simulink library "DiSC_ToolboxOpal_V12"  (R2012b)
settings: Solver=ode45  StartTime=0.0  StopTime=10.0  RelTol=1e-3
undefined symbols (not defined in the file or in its folder): SamplingTime
(part 3 of 5)

== system DiSC_ToolboxOpal_V12/scAsset ==
  In1 : Inport
  In2 : Inport  Port=2
  In3 : Inport  Port=3
  In4 : Inport  Port=4
  MATLAB Function : MATLAB Function  TreatAsAtomicUnit=on
  Out1 : Outport
  wires:
  MATLAB Function/1(q) -> Out1/1
  In4/1 -> MATLAB Function/4(t)
  In1/1 -> MATLAB Function/1(v)
  In2/1 -> MATLAB Function/2(qRef)
  In3/1 -> MATLAB Function/3(vRef)

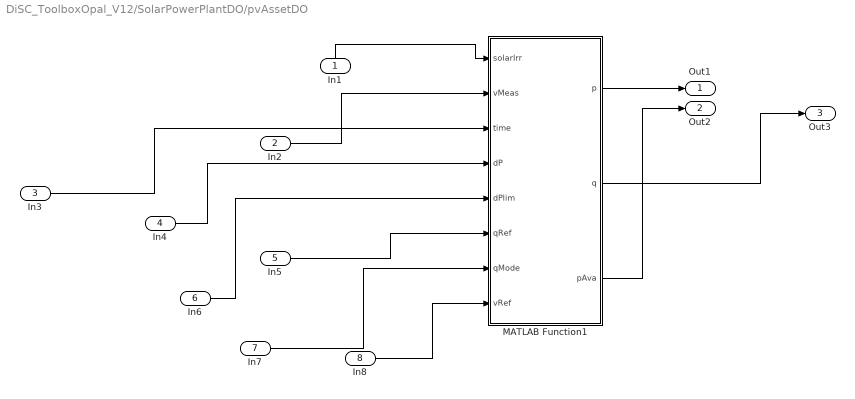
== system DiSC_ToolboxOpal_V12/SolarPowerPlantDO/pvAssetDO ==
  In1 : Inport
  In2 : Inport  Port=2
  In3 : Inport  Port=3
  In4 : Inport  Port=4
  In5 : Inport  Port=5
  In6 : Inport  Port=6
  In7 : Inport  Port=7
  In8 : Inport  Port=8
  MATLAB Function1 : MATLAB Function  TreatAsAtomicUnit=on
  Out1 : Outport
  Out2 : Outport  Port=2
  Out3 : Outport  Port=3
  wires:
  MATLAB Function1/3(pAva) -> Out2/1
  In5/1 -> MATLAB Function1/6(qRef)
  MATLAB Function1/1(p) -> Out1/1
  In2/1 -> MATLAB Function1/2(vMeas)
  In4/1 -> MATLAB Function1/4(dP)
  In6/1 -> MATLAB Function1/5(dPlim)
  In3/1 -> MATLAB Function1/3(time)
  In1/1 -> MATLAB Function1/1(solarIrr)
  MATLAB Function1/2(q) -> Out3/1
  In8/1 -> MATLAB Function1/8(vRef)
  In7/1 -> MATLAB Function1/7(qMode)

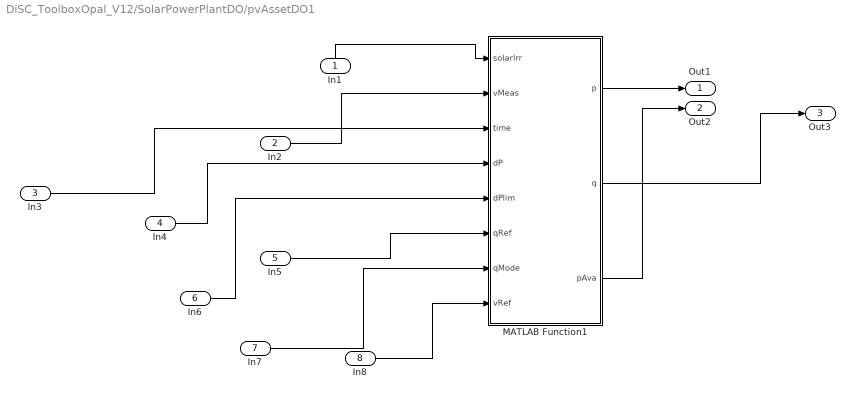
== system DiSC_ToolboxOpal_V12/SolarPowerPlantDO/pvAssetDO1 ==
  In1 : Inport
  In2 : Inport  Port=2
  In3 : Inport  Port=3
  In4 : Inport  Port=4
  In5 : Inport  Port=5
  In6 : Inport  Port=6
  In7 : Inport  Port=7
  In8 : Inport  Port=8
  MATLAB Function1 : MATLAB Function  TreatAsAtomicUnit=on
  Out1 : Outport
  Out2 : Outport  Port=2
  Out3 : Outport  Port=3
  wires:
  MATLAB Function1/3(pAva) -> Out2/1
  In5/1 -> MATLAB Function1/6(qRef)
  MATLAB Function1/1(p) -> Out1/1
  In2/1 -> MATLAB Function1/2(vMeas)
  In4/1 -> MATLAB Function1/4(dP)
  In6/1 -> MATLAB Function1/5(dPlim)
  In3/1 -> MATLAB Function1/3(time)
  In1/1 -> MATLAB Function1/1(solarIrr)
  MATLAB Function1/2(q) -> Out3/1
  In8/1 -> MATLAB Function1/8(vRef)
  In7/1 -> MATLAB Function1/7(qMode)

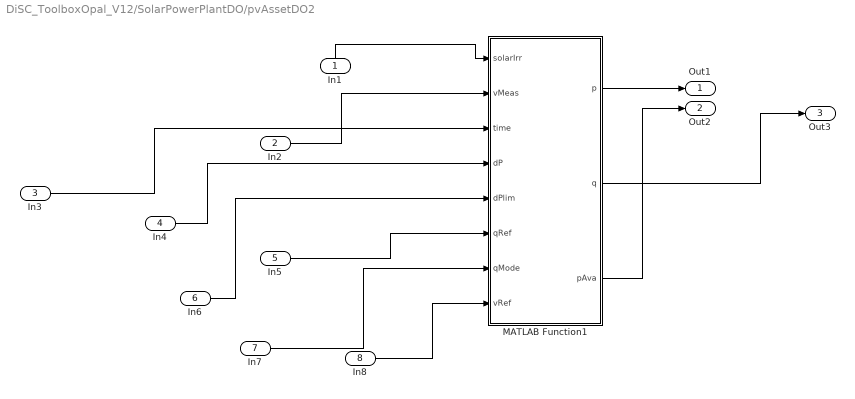
== system DiSC_ToolboxOpal_V12/SolarPowerPlantDO/pvAssetDO2 ==
  In1 : Inport
  In2 : Inport  Port=2
  In3 : Inport  Port=3
  In4 : Inport  Port=4
  In5 : Inport  Port=5
  In6 : Inport  Port=6
  In7 : Inport  Port=7
  In8 : Inport  Port=8
  MATLAB Function1 : MATLAB Function  TreatAsAtomicUnit=on
  Out1 : Outport
  Out2 : Outport  Port=2
  Out3 : Outport  Port=3
  wires:
  MATLAB Function1/3(pAva) -> Out2/1
  In5/1 -> MATLAB Function1/6(qRef)
  MATLAB Function1/1(p) -> Out1/1
  In2/1 -> MATLAB Function1/2(vMeas)
  In4/1 -> MATLAB Function1/4(dP)
  In6/1 -> MATLAB Function1/5(dPlim)
  In3/1 -> MATLAB Function1/3(time)
  In1/1 -> MATLAB Function1/1(solarIrr)
  MATLAB Function1/2(q) -> Out3/1
  In8/1 -> MATLAB Function1/8(vRef)
  In7/1 -> MATLAB Function1/7(qMode)

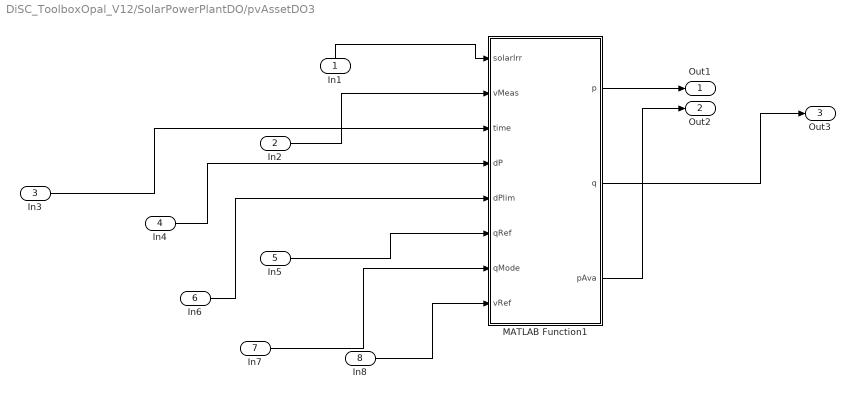
== system DiSC_ToolboxOpal_V12/SolarPowerPlantDO/pvAssetDO3 ==
  In1 : Inport
  In2 : Inport  Port=2
  In3 : Inport  Port=3
  In4 : Inport  Port=4
  In5 : Inport  Port=5
  In6 : Inport  Port=6
  In7 : Inport  Port=7
  In8 : Inport  Port=8
  MATLAB Function1 : MATLAB Function  TreatAsAtomicUnit=on
  Out1 : Outport
  Out2 : Outport  Port=2
  Out3 : Outport  Port=3
  wires:
  MATLAB Function1/3(pAva) -> Out2/1
  In5/1 -> MATLAB Function1/6(qRef)
  MATLAB Function1/1(p) -> Out1/1
  In2/1 -> MATLAB Function1/2(vMeas)
  In4/1 -> MATLAB Function1/4(dP)
  In6/1 -> MATLAB Function1/5(dPlim)
  In3/1 -> MATLAB Function1/3(time)
  In1/1 -> MATLAB Function1/1(solarIrr)
  MATLAB Function1/2(q) -> Out3/1
  In8/1 -> MATLAB Function1/8(vRef)
  In7/1 -> MATLAB Function1/7(qMode)

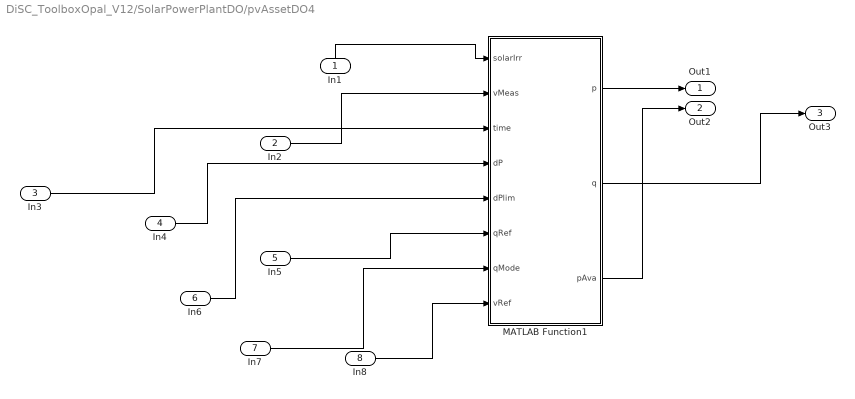
== system DiSC_ToolboxOpal_V12/SolarPowerPlantDO/pvAssetDO4 ==
  In1 : Inport
  In2 : Inport  Port=2
  In3 : Inport  Port=3
  In4 : Inport  Port=4
  In5 : Inport  Port=5
  In6 : Inport  Port=6
  In7 : Inport  Port=7
  In8 : Inport  Port=8
  MATLAB Function1 : MATLAB Function  TreatAsAtomicUnit=on
  Out1 : Outport
  Out2 : Outport  Port=2
  Out3 : Outport  Port=3
  wires:
  MATLAB Function1/3(pAva) -> Out2/1
  In5/1 -> MATLAB Function1/6(qRef)
  MATLAB Function1/1(p) -> Out1/1
  In2/1 -> MATLAB Function1/2(vMeas)
  In4/1 -> MATLAB Function1/4(dP)
  In6/1 -> MATLAB Function1/5(dPlim)
  In3/1 -> MATLAB Function1/3(time)
  In1/1 -> MATLAB Function1/1(solarIrr)
  MATLAB Function1/2(q) -> Out3/1
  In8/1 -> MATLAB Function1/8(vRef)
  In7/1 -> MATLAB Function1/7(qMode)

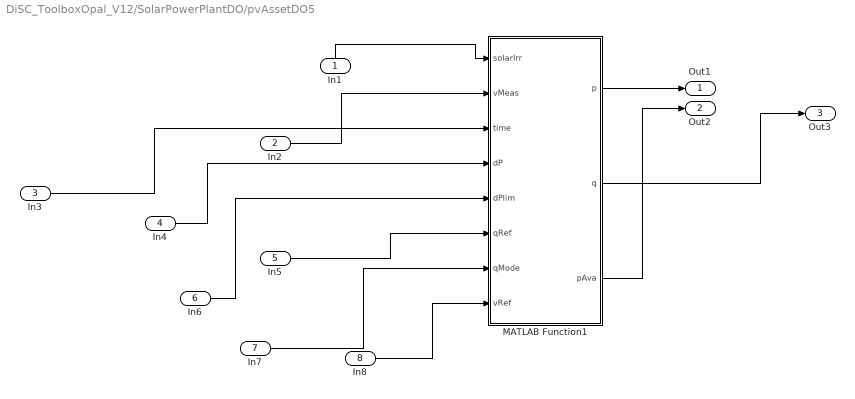
== system DiSC_ToolboxOpal_V12/SolarPowerPlantDO/pvAssetDO5 ==
  In1 : Inport
  In2 : Inport  Port=2
  In3 : Inport  Port=3
  In4 : Inport  Port=4
  In5 : Inport  Port=5
  In6 : Inport  Port=6
  In7 : Inport  Port=7
  In8 : Inport  Port=8
  MATLAB Function1 : MATLAB Function  TreatAsAtomicUnit=on
  Out1 : Outport
  Out2 : Outport  Port=2
  Out3 : Outport  Port=3
  wires:
  MATLAB Function1/3(pAva) -> Out2/1
  In5/1 -> MATLAB Function1/6(qRef)
  MATLAB Function1/1(p) -> Out1/1
  In2/1 -> MATLAB Function1/2(vMeas)
  In4/1 -> MATLAB Function1/4(dP)
  In6/1 -> MATLAB Function1/5(dPlim)
  In3/1 -> MATLAB Function1/3(time)
  In1/1 -> MATLAB Function1/1(solarIrr)
  MATLAB Function1/2(q) -> Out3/1
  In8/1 -> MATLAB Function1/8(vRef)
  In7/1 -> MATLAB Function1/7(qMode)

== system DiSC_ToolboxOpal_V12/WindPowerPlant/wtAssetDO ==
  In1 : Inport
  In2 : Inport  Port=2
  In3 : Inport  Port=3
  In4 : Inport  Port=4
  In5 : Inport  Port=5
  In6 : Inport  Port=6
  In7 : Inport  Port=7
  In8 : Inport  Port=8
  MATLAB Function : MATLAB Function  TreatAsAtomicUnit=on
  Out1 : Outport
  Out2 : Outport  Port=2
  Out3 : Outport  Port=3
  wires:
  In1/1 -> MATLAB Function/1(wind)
  MATLAB Function/3(pAva) -> Out2/1
  In4/1 -> MATLAB Function/4(dPlim)
  MATLAB Function/2(q) -> Out3/1
  In2/1 -> MATLAB Function/2(vMeas)
  In3/1 -> MATLAB Function/3(dP)
  MATLAB Function/1(p) -> Out1/1
  In7/1 -> MATLAB Function/7(vRef)
  In6/1 -> MATLAB Function/6(qMode)
  In5/1 -> MATLAB Function/5(qRef)
  In8/1 -> MATLAB Function/8(time)

== system DiSC_ToolboxOpal_V12/WindPowerPlant/wtAssetDO1 ==
  In1 : Inport
  In2 : Inport  Port=2
  In3 : Inport  Port=3
  In4 : Inport  Port=4
  In5 : Inport  Port=5
  In6 : Inport  Port=6
  In7 : Inport  Port=7
  In8 : Inport  Port=8
  MATLAB Function : MATLAB Function  TreatAsAtomicUnit=on
  Out1 : Outport
  Out2 : Outport  Port=2
  Out3 : Outport  Port=3
  wires:
  In1/1 -> MATLAB Function/1(wind)
  MATLAB Function/3(pAva) -> Out2/1
  In4/1 -> MATLAB Function/4(dPlim)
  MATLAB Function/2(q) -> Out3/1
  In2/1 -> MATLAB Function/2(vMeas)
  In3/1 -> MATLAB Function/3(dP)
  MATLAB Function/1(p) -> Out1/1
  In7/1 -> MATLAB Function/7(vRef)
  In6/1 -> MATLAB Function/6(qMode)
  In5/1 -> MATLAB Function/5(qRef)
  In8/1 -> MATLAB Function/8(time)

== system DiSC_ToolboxOpal_V12/WindPowerPlant/wtAssetDO2 ==
  In1 : Inport
  In2 : Inport  Port=2
  In3 : Inport  Port=3
  In4 : Inport  Port=4
  In5 : Inport  Port=5
  In6 : Inport  Port=6
  In7 : Inport  Port=7
  In8 : Inport  Port=8
  MATLAB Function : MATLAB Function  TreatAsAtomicUnit=on
  Out1 : Outport
  Out2 : Outport  Port=2
  Out3 : Outport  Port=3
  wires:
  In1/1 -> MATLAB Function/1(wind)
  MATLAB Function/3(pAva) -> Out2/1
  In4/1 -> MATLAB Function/4(dPlim)
  MATLAB Function/2(q) -> Out3/1
  In2/1 -> MATLAB Function/2(vMeas)
  In3/1 -> MATLAB Function/3(dP)
  MATLAB Function/1(p) -> Out1/1
  In7/1 -> MATLAB Function/7(vRef)
  In6/1 -> MATLAB Function/6(qMode)
  In5/1 -> MATLAB Function/5(qRef)
  In8/1 -> MATLAB Function/8(time)

== system DiSC_ToolboxOpal_V12/WindPowerPlant/wtAssetDO3 ==
  In1 : Inport
  In2 : Inport  Port=2
  In3 : Inport  Port=3
  In4 : Inport  Port=4
  In5 : Inport  Port=5
  In6 : Inport  Port=6
  In7 : Inport  Port=7
  In8 : Inport  Port=8
  MATLAB Function : MATLAB Function  TreatAsAtomicUnit=on
  Out1 : Outport
  Out2 : Outport  Port=2
  Out3 : Outport  Port=3
  wires:
  In1/1 -> MATLAB Function/1(wind)
  MATLAB Function/3(pAva) -> Out2/1
  In4/1 -> MATLAB Function/4(dPlim)
  MATLAB Function/2(q) -> Out3/1
  In2/1 -> MATLAB Function/2(vMeas)
  In3/1 -> MATLAB Function/3(dP)
  MATLAB Function/1(p) -> Out1/1
  In7/1 -> MATLAB Function/7(vRef)
  In6/1 -> MATLAB Function/6(qMode)
  In5/1 -> MATLAB Function/5(qRef)
  In8/1 -> MATLAB Function/8(time)

== system DiSC_ToolboxOpal_V12/WindPowerPlant/wtAssetDO4 ==
  In1 : Inport
  In2 : Inport  Port=2
  In3 : Inport  Port=3
  In4 : Inport  Port=4
  In5 : Inport  Port=5
  In6 : Inport  Port=6
  In7 : Inport  Port=7
  In8 : Inport  Port=8
  MATLAB Function : MATLAB Function  TreatAsAtomicUnit=on
  Out1 : Outport
  Out2 : Outport  Port=2
  Out3 : Outport  Port=3
  wires:
  In1/1 -> MATLAB Function/1(wind)
  MATLAB Function/3(pAva) -> Out2/1
  In4/1 -> MATLAB Function/4(dPlim)
  MATLAB Function/2(q) -> Out3/1
  In2/1 -> MATLAB Function/2(vMeas)
  In3/1 -> MATLAB Function/3(dP)
  MATLAB Function/1(p) -> Out1/1
  In7/1 -> MATLAB Function/7(vRef)
  In6/1 -> MATLAB Function/6(qMode)
  In5/1 -> MATLAB Function/5(qRef)
  In8/1 -> MATLAB Function/8(time)

== system DiSC_ToolboxOpal_V12/WindPowerPlant/wtAssetDO5 ==
  In1 : Inport
  In2 : Inport  Port=2
  In3 : Inport  Port=3
  In4 : Inport  Port=4
  In5 : Inport  Port=5
  In6 : Inport  Port=6
  In7 : Inport  Port=7
  In8 : Inport  Port=8
  MATLAB Function : MATLAB Function  TreatAsAtomicUnit=on
  Out1 : Outport
  Out2 : Outport  Port=2
  Out3 : Outport  Port=3
  wires:
  In1/1 -> MATLAB Function/1(wind)
  MATLAB Function/3(pAva) -> Out2/1
  In4/1 -> MATLAB Function/4(dPlim)
  MATLAB Function/2(q) -> Out3/1
  In2/1 -> MATLAB Function/2(vMeas)
  In3/1 -> MATLAB Function/3(dP)
  MATLAB Function/1(p) -> Out1/1
  In7/1 -> MATLAB Function/7(vRef)
  In6/1 -> MATLAB Function/6(qMode)
  In5/1 -> MATLAB Function/5(qRef)
  In8/1 -> MATLAB Function/8(time)

== matlab function DiSC_ToolboxOpal_V12/ElectricVehicle/MATLAB Function ==
  data: day input; p output; vMeas input; pRef input; pMode input; qRef input; qMode input; vRef input; time input; seed input; q output; e output; away output
function [p,q,e,away] = evAssetDO(day,vMeas,pRef,pMode,qRef,qMode,vRef,time,seed)
%#codegen
  % evAsset implements a simple electrical vehical mobility- and battery model in Simulink.
    %   The active power consumption of the battery charging cycle can be
    %   controlled when ever the electrical vehical is available at
    %   a household charging spot.
    %   To simulate when the electrical vehical is available data from the
    %   National Travel Survey from Great Britain is used.
    %
    %   To model the battery a simple first order model of an energy
    %   storages is used. The batterys state of charges, when arriving at a
    %   charging station/spot, is dependent on the trip the car has conducted.
    %
    %
    % Revision:
    % 16-07-2014, C.E. Sloth and R. Pedersen, Aalborg University. Notes:
    % 29-11-2014, R. Olsen/M. Kemal, Aalborg University (Simulink)
    % 20-06-2015, F. Iov/M. Kemal, Aalborg University (Simulink toolbox for OPAL)
            % Input:
            %   - k [-], is the sample number.
            %   - day [day number], is the day of the year 1-365.
            %   - v [-], is the voltage at the connection point.
            %   - pRef [W], is the reference to active power.
            %   - qRef [VAR], is the reference to reactive power.
            %   - vRef [V], is the voltage reference.
            %
            % Output:
            %   - p [W], is the active power output.
            %   - q [VAR], is the reactive power output.
            %   - e [J], is the EV batery energy level.
            %   - away [-]. Indicates if the EV is available for charging.
            
            % If day changes calculate when EV is away from home and how
            % much the state of charge has changed.
            
        %properties    
        param.vBase = 20e3;               % Voltage base [V].
        param.pRated = 6e6;               % Rated output power [W].
        param.sMax = 3e6;                 % Maximum apparent power [VA].
        param.pRate = 1000;                 % Constraint on power rate of change [W/s].
        param.PF = 1;                     % Power factor [-].
        param.a = 1;                      % Drain rate of battery [-].
        param.eta = 1;                    % Efficiency of battery [-].
        param.avgMileage = 2;             % Average mileage [% battery/mile].
        param.eRated = 65e3*60*60;        % Battery capacity [J].
        param.Ts = 60;  
        
       %variables
       persistent var;
       if isempty(var) 
        var.eOld = 0;                   % Place holder for battery state [J].
        var.pOld = 0;                   % Power consumption last sample [W].
        var.pMode = 0;                  % Indicates which control mode the charging of the EV is in [-].
        var.qMode = 0;                  % Reactive power control mode [-].
        
        % Modified data based on Table NTS0503
        var.toEducation = [0 0 0 0 0 0 0 7 40 2 1 0 0 0 0 0 0 0 0 0 0 0 0 0];
        var.fromEducation = [0 0 0 0 0 0 0 0 0 0 0 1 2 2 3 32 5 2 1 0 0 0 0 0];
        var.toShopping =    [0 0 0 0 0 0 0 1 2 5 7 7 6 4.5 4.5 3 3 2 2 2 1 0 0 0];
        var.fromShopping =  [0 0 0 0 0 0 0 0 1 3 5 6 5 5 5 5 4 4 3 2 1 1 0 0];
        var.toCommute =   [0 0 0 0 0 3 7 16 15 4 2 2 1 0 0 0 0 0 0 0 0 0 0 0];
        var.fromCommute = [0 0 0 0 0 0 0 0 0 0 0 0 2 3 3 4 9 15 7 2 2 1 1 1];
        var.businessStart = [0 0 0 0 0.5 1 3 7 10 8 7 7 7 7 7 8 9 8 4 2 2 1 1 0.5];
        var.toBusiness =   [0 0 0 0 0.5 1 3 7 10 8 6 5 3.5 2 2 1 1 0 0 0 0 0 0 0];
        var.fromBusiness = [0 0 0 0 0   0 0 0 0  0 1 2 3.5 5 5 7 8 8 4 2 2 1 1 0.5];
        var.toEscortEducation =   [0 0 0 0 0 0 0 3 36 7 0 2 2 0 0 0 0 0 0 0 0 0 0 0];
        var.fromEscortEducation = [0 0 0 0 0 0 0 0 0 0 0 0 0 1 9 33 4 2 1 0 0 0 0 0];
        var.toOtherPersonal =   [0 0 0 0 0 0 1 4 8 8 7 7 6 4 2 1 1 1 0 0 0 0 0 0];
        var.fromOtherPersonal = [0 0 0 0 0 0 0 0 0 0 1 1 2 3 5 7 8 7 6 4 2 2 1 1];
        var.toVisit =   [0 0 0 0 0 0 1 1 2 4 5 6 6 5 4 4 3 3 3 2 1 0 0 0];
        var.fromVisit = [0 0 0 0 0 0 0 0 0 0 0 0 0 1 2 4 5 6 7 8 5 5 4 3];
        var.toHoliday =    [0 0 0 0 0 0 2 4 5 7 8 6 3 3 3 2 2 2 2 1 0 0 0 0];
        var.fromHoliday =  [0 0 0 0 0 0 0 0 0 0 1 3 3 4 5 7 7 5 5 4 3 2 1 1];
        
        % CDFs of mobility model
        var.toCommutingCDF=zeros(1,24);
        var.fromCommutingCDF=zeros(1,24);
        var.toBusinessCDF=zeros(1,24);
        var.fromBusinessCDF=zeros(1,24);
        var.toEducationCDF=zeros(1,24);
        var.fromEducationCDF=zeros(1,24);
        var.toEscortEducationCDF=zeros(1,24);
        var.fromEscortEducationCDF=zeros(1,24);
        var.toShoppingCDF=zeros(1,24);
        var.fromShoppingCDF=zeros(1,24);
        var.toPersonalBusinessOtherEscortCDF=zeros(1,24);
        var.fromPersonalBusinessOtherEscortCDF=zeros(1,24);
        var.toVisitFriendsSportCDF=zeros(1,24);
        var.fromVisitFriendsSportCDF=zeros(1,24);
        var.toHolidayCDF=zeros(1,24);
        var.fromHolidayCDF=zeros(1,24);

        var.away=zeros(1,26);                     % [-]. Indicates if vehicle is home and ready for charging, 0 = at home and 1 = away
        var.dSOC = zeros(1,24);                   % [%]. Change in battery state of charge

        
        % Average trip length in miles Table NTS0405
        % We only consider round-trips; hence, the length from the data is multiplied by two
        var.CommutingLength = 9*2;
        var.BusinessLength = 19.6*2;
        var.EducationLength = 3.4*2;
        var.EscortEducationLength = 2.4*2;
        var.ShoppingLength = 4.4*2;
        var.OtherEscortLength = 5.5*2;
        var.PersonalBusinessLength = 5.2*2;
        var.VisitFriendsPrivateHomeLength = 10.2*2;
        var.VisitFriendsElsewhereLength = 6.4*2;
        % Sport and Entertainment separated in NTS0405; hence, average is used
        var.SportLength = (7.6+6.4)/2*2;
        % Holiday and Day trip separated in NTS0405; hence, average is used
        var.HolidayLength = (43.3+13.1)/2*2;
        
        % parameters
        var.daysPerYear = 365;
        var.individualDayOfWeekPerYear = 1;
        
        % Round-trip rates as car driver by day of weak
        % Probability of being driver of car/van for trip (based on Table NTS0409)
        var.CommutingCarDriverProb = 84/146;
        var.BusinessCarDriverProb = 22/31;
        var.EducationOrEduEscortCarDriverProb = 26/116;
        var.ShoppingCarDriverProb = 85/189;
        var.OtherEscortCarDriverProb = 50/87;
        var.PersonalBusinessCarDriverProb = 41/94;
        var.LeisureCarDriverProb = 93/248;
        
        % Trip rates by day of weak from Table NTS0504 (We only consider round-trips; hence, the number of trips from the data is divided by two)
        var.CommutingPerYear = [26  28 28 28 26 9 5]/2;
        var.BusinessPerYear = [5  6 6 6 5 2 1]/2;
        var.EducationPerYear = [12  12 13 12 11 0 0]/2;
        var.EscortEducationPerYear = [9 9 9 9 9 0 0]/2;
        var.ShoppingPerYear = [25 24 25 26 29 42 23]/2;
        var.OtherEscortPerYear = [13 14 14 13 14 14 10]/2;
        var.PersonalBusinessPerYear = [15 16 16 16 15 9 11]/2;
        var.VisitFriendsPrivateHomePerYear = [12 12 13 13 14 20 21]/2;
        var.VisitFriendsElsewherePerYear = [4 4 5 6 8 10 9]/2;
        var.SportPerYear = [8 9 10 9 8 12 8]/2;
        var.HolidayPerYear = [5 5 6 6 6 7 8]/2;
        
        % Mobility model
        var.dayOld = -1;                % [-]. Used to check if day has changed
        var.temp = 0;                   % [-]. Flag used for the mobility model
        var.h = 2;                      % [-]. Sample of the day

        %Used for caching
        var.p_c=0;
        var.q_c=0;
        var.e_c=0;
        var.away_c=0;
        var.t_c=0;
        var.k=0; 
       end
        
         % Compute parameters
            var.eOld = param.eRated;
            var.individualDayOfWeekPerYear = var.daysPerYear/7;
            
            % Setup CDFs of mobility model
            [var.toCommutingCDF, var.fromCommutingCDF] = getToFromCDFs(var,var.toCommute,var.fromCommute);
            [var.toBusinessCDF, var.fromBusinessCDF] = getToFromCDFs(var,var.toBusiness,var.fromBusiness);
            [var.toEducationCDF, var.fromEducationCDF] = getToFromCDFs(var,var.toEducation,var.fromEducation);
            [var.toEscortEducationCDF, var.fromEscortEducationCDF] = getToFromCDFs(var,var.toEscortEducation,var.fromEscortEducation);
            [var.toShoppingCDF, var.fromShoppingCDF] = getToFromCDFs(var,var.toShopping,var.fromShopping);
            [var.toPersonalBusinessOtherEscortCDF, var.fromPersonalBusinessOtherEscortCDF] = getToFromCDFs(var,var.toOtherPersonal,var.fromOtherPersonal);
            [var.toVisitFriendsSportCDF, var.fromVisitFriendsSportCDF] = getToFromCDFs(var,var.toVisit,var.fromVisit);
            [var.toHolidayCDF, var.fromHolidayCDF] = getToFromCDFs(var,var.toHoliday,var.fromHoliday);
            
            % Round-trip rates as car driver (note that probability of car by purpose is only available for groups of purposes)
            var.CommutingPerYear = var.CommutingPerYear*var.CommutingCarDriverProb;
            var.BusinessPerYear = var.BusinessPerYear*var.BusinessCarDriverProb; 
            var.EducationPerYear = var.EducationPerYear*var.EducationOrEduEscortCarDriverProb; 
            var.EscortEducationPerYear = var.EscortEducationPerYear*var.EducationOrEduEscortCarDriverProb; 
            var.ShoppingPerYear = var.ShoppingPerYear*var.ShoppingCarDriverProb; 
            var.OtherEscortPerYear = var.OtherEscortPerYear*var.OtherEscortCarDriverProb; 
            var.PersonalBusinessPerYear = var.PersonalBusinessPerYear*var.PersonalBusinessCarDriverProb; 
            var.VisitFriendsPrivateHomePerYear = var.VisitFriendsPrivateHomePerYear*var.LeisureCarDriverProb; 
            var.VisitFriendsElsewherePerYear = var.VisitFriendsElsewherePerYear*var.LeisureCarDriverProb; 
            var.SportPerYear = var.SportPerYear*var.LeisureCarDriverProb; 
            var.HolidayPerYear = var.HolidayPerYear*var.LeisureCarDriverProb; 
            
             % Implement algorithm. 
            if (param.Ts>0)
               if (time>(var.t_c+param.Ts))
                 
                   [p_c,q_c,e_c,away_c,varNew] = sampleEV(param,var,day,vMeas,pRef,qRef,vRef,seed);
                   var=varNew;
                   var.p_c=p_c;
                   var.q_c=q_c;
                   var.e_c=e_c;
                   var.away_c=away_c;      
                   var.t_c=time;
                   var.k=var.k+1;
                   var.pMode = pMode;
                   var.qMode = qMode;
               end
               p=var.p_c;
               q=var.q_c;
               e=var.e_c;
               away=var.away_c;
            else
                 [p,q,e,away,varNew] = sampleEV(param,var,day,vMeas,pRef,qRef,vRef,seed);
                 var=varNew;
                 var.k=var.k+1;
            end
end

== matlab function DiSC_ToolboxOpal_V12/CapBank/MATLAB Function ==
  data: q output; v input; vRef input; uRef input; setQmode input; t input; day input
function q = cbAssetDO(v,vRef,uRef,setQmode,t,day)
%#codegen
    % A simulink version of cbAsset module using embedded matlab function
    % block on Simulink
    %   The cbAsset can be controlled to inject reactive power into the
    %   grid in steps. It is characterized by having a number of steps and
    %   a reactive output per step (i.e., it can inject from 0 - Qmax in 
    %   N steps). 
    %   
    %   
    % Revision:
    % 15-10-2014, R. Pedersen, Aalborg University. Notes:
    % 29-11-2014, R. Olsen/M. Kemal, Aalborg University (Simulink)
    % 20-06-2015, F. Iov/M. Kemal, Aalborg University (Simulink toolbox for OPAL)

        % Input:
            %   - v [V], is the voltage at the connection point.
            %   - qRef [VAR], is the reference to active power.
            %   - vRef [V], is the voltage reference for the droop control.
            %   - uRef [V], is the tap reference 
            %   - SetQmode will set the reactive power control  mode 
            %
            % Output:
            %   - q [VAR], is the reactive power output   
    
 %    parameters

        param.sBase = 400e3;          % Complex power base [VA].               
        param.vBase = 0.4e3;          % Voltage base [V].              
        param.qMax = 50e3;            % Maximum reactive power output [VAR].     
        param.Ts = 60;                % Sampling time [sec].      
        param.onPU = false;           % Simulate on per unit. 
        param.nStepPrDay = 15;        % Maximum number of steps per day [-]. 
        param.tMin = 10*60;           % Minimum time between steps [s]. 
        param.nSteps = 10;            % Number of steps to reach qMax [-]. 
        param.vHyst = 0.05;           % Hysterisis limit for voltage control [%]. 
 
%   variables                 
     persistent var;
     if isempty(var) 
        var.avgFilterTime = 10*60;      % Time window of the moving average filter [sec].    
        var.avgFilterBuf = ones(10,1);

         
        var.stepChDay = 0;          % Number of steps that has occured in a day [-].
        var.dayOld = -1;            % Used to check if day has changed [-].
        var.stepOk = 1;             % Flag indicating if step is allowed (1=yes, 0=no) [-].  
        var.stepTimer = 0;          % Timer indicating if a step is allowed, i.e., the timer must be greater than kMin to apply change [-].
        var.stepPos = 0;            % Position of the capacitor bank (how many capacitors are coupled in) [-].
        var.qStep=0;           % Reactive power per step [VAR].
        var.kMin= 0;                 % Minimum number of samples between steps [-].
        var.qMode = 1;              % Mode for control (0 = follow reference, 1 = voltage control) [-]. 
        var.t_c=0;  %Caching time
        var.q_c=0;  %Cached q value        
        var.k=0;                    %Sample nr.
     end
    
%             Check if the simulation is on per unit
                if param.onPU == true
                    vAvgFilterTemp = 1;
                else
                    vAvgFilterTemp = param.vBase;
                    
                end   
                
                % Compute reactive power per step
                var.qStep = param.qMax/param.nSteps;

                % Compute minimum samples between capacitor bank step
                var.kMin = ceil(param.tMin/param.Ts);
                var.avgFilterBuf = vAvgFilterTemp*var.avgFilterBuf;
               
                
                % Implement algorithm.
             if (param.Ts>0)
                if (t>(var.t_c+param.Ts))
                   [q_c,varNew] = sampleCB(param,var,v,vRef,uRef,day);
                   var=varNew;
                   var.q_c=q_c;
                   var.t_c=t;
                   var.k=var.k+1;
                   var.qMode = setQmode;
                   
                end
                q=var.q_c;           
            else
                [q,varNew]=sampleCB(param,var,v,vRef,uRef,day);
                varNew=var;
                var.k=var.k+1;
                var.qMode = setQmode;
            end               
              
 end

== matlab function DiSC_ToolboxOpal_V12/EnergyStorage/MATLAB Function ==
  data: vMeas input; p output; pRef input; pMode input; qRef input; qMode input; vRef input; time input; q output; e output
function [p,q,e] = esAssetDO(vMeas,pRef,pMode,qRef,qMode,vRef, time)
%#codegen
    % A Simulink model of esAsset for Simulink using embedded matlab
    % function
    % esAsset implements a simple controllable energy storage.
    %   The esAsset can be set to consume active power or inject active
    %   power. The energy storage consumes reactive power with a constant
    %   power factor. The energy storage can also be set to do voltage
    %   droop control.
    %   
    %   
    % Revision:
    % 23-06-2014, R. Pedersen, Aalborg University. Notes:
    % 29-11-2014, R. Olsen/M. Kemal, Aalborg University (Simulink)
    % 20-06-2015, F. Iov/M. Kemal, Aalborg University (Simulink toolbox for OPAL)
    
            % Input:
            %   - v, is the voltage at the connection point.
            %   - pRef, is the reference to active power.
            %   - vRef, is the voltage reference for the droop control
            %
            % Output:
            %   - p [W], is the active power consumption
            %   - q [VAR], is the reactive power output
            %   - e [J], is the energy storage energy level
            
%     parameters         
        param.vBase = 400;            % Voltage base [V].    
        param.pRatedMax = 10e3;       % Rated power consumption [W].    
        param.pRatedMin = -10e3;       % Rated power output [W].     
        param.pRate = 600;             % Constraint on power rate of change [W/sec].     
        param.sMax = 10e3;            % Maximum apparent power [VA].    
        param.PF = 1;                 % Power factor [-].    
        param.eRated = 100e6;          % Rated energy level [J].    
       
        param.Ts = 60;                % Sampling time [sec].     
        param.a = 1;                  % Energy storage drain rate [-].     
        param.etaIn = 0.7;              % Energy storage effeciency when charging [-].     
        param.etaOut = 0.9;             % Energy storage efficiency when discharging [-].
        
         %variables 
        persistent var;
        if isempty(var)  
         var.avgFilterTime = 10*60;                   % [s]. Time window of the moving average filter
         var.avgFilterBuf = ones(ceil(10*60/60),1);   %Memory allocation to make it compatible with simulink % [-]. Buffer for the moving average filter
         var.pMode = 1;              % Mode for the control of active power [-].     
         var.qMode = 1;              % Mode for the control of reactive power [-]. 
       
         var.pOld = 0;               % Placeholder for power. Used for rate constraint [W].     
         var.eOld = 0;               % Placeholder for energy level [J].     
         var.t_c=0;  %Caching time
         var.q_c=0;  %Cached q value
         var.p_c=0;  %Cached p value
         var.e_c=0;  %Cached e value
         var.k=0;    %Sample nr.y = u;
        end
       
            % Setup the buffer for the moving average filter
            var.avgFilterBuf = param.vBase*var.avgFilterBuf;
            

            if (param.Ts>0)
               if (time>(var.t_c+param.Ts))
                   [p,q,e,varNew] = sampleES(param,var,vMeas,pRef,qRef,vRef);
                   var=varNew;
                   var.p_c=p;
                   var.q_c=q;
                   var.e_c=e;
                   var.t_c=time;
                   var.k=varNew.k+1;
                   var.qMode = qMode;
                   var.pMode = pMode;
               end
               p=var.p_c;
               q=var.q_c;
               e=var.e_c;   
                
            else
                [p,q,e,varNew] = sampleES(param,var,vMeas,pRef,qRef,vRef);
                var=varNew;
                var.k=var.k+1;
            end
end

== matlab function DiSC_ToolboxOpal_V12/CloudCover/MATLAB Function1 ==
  data: mean input; cc output; var input; x input
function cc = cloudCoverDO(mean,var,x)
%#codegen
    % A Simulink version of the CloudCover model using
   %MATLAB embedded block  for OPAL-RT
    %
    %   The cloud cover model can be used to investigate the behavior
    %   of e.g., photovoltaic systems. This model can be used together with
    %   the solar irradiance model.
    %
    %   The model is based on the work by
    %   Heinriich Morf (1998-2013)
    %
    % Revision:
    % R. Pedersen, Aalborg University.
    % 29-11-2014, R. Olsen/M. Kemal, Aalborg University (Simulink)
    % 20-06-2015, F. Iov/M. Kemal, Aalborg University (Simulink toolbox for OPAL)
    
    %parameter properties        
        % For cloud cover model (cc)
        param.M = 50;         % number of observation points [-]      
        param.Aobs = 1;       % observed area (can be set to 1 if unknown) [m^2] 
        
    %variable properties
    
     persistent vari;
     if isempty(vari)         
    
        vari.mean = 0.3;  % [-], mean of cloud cover
        vari.A1_m = 0;       % [m^2], mean of covered area
        vari.A0_m = 1;       % [m^2], mean of non-covered area
        vari.P = zeros(2,2);   % [-], transition probability matrix
       
        vari.ccOld=zeros(50,1);         % [-], array of placeholder for cc, N long
        vari.n = 1;
        vari.var = 0.1567;           % [-], variance of cloud cover
        
     end
     
                 % Implement algorithm. 
            
            variNew=setMeanVarInternal(param,vari,mean,var,x);
            vari=variNew;
            [cc,variNew] = sampleCc(param,vari);
             vari=variNew;

            
           
           
end

== matlab function DiSC_ToolboxOpal_V12/PV System/MATLAB Function1 ==
  data: solarIrr input; p output; vMeas input; time input; dP input; dPlim input; qRef input; qMode input; vRef input; q output; pAva output
function [p,q,pAva] = pvAssetDO(solarIrr,vMeas,time,dP,dPlim,qRef,qMode,vRef)

%#codegen
%pvAssetDO implements a simple P,Q controllable solar PV system using MATLAB embedded function.
    %   The pvAsset can be set to follow an active power reference, output
    %   maximum power available or derate power. It can also, at the same
    %   time be set to follow a reactive power reference, output the
    %   minimum reactive power according to the power factor or try to keep
    %   a voltage reference in the coupling point by controlling reactive
    %   power output.
    %   
    %   
    % Revision:
    % 19-06-2014, R. Pedersen, Aalborg University. Notes:
    % R. Pedersen 11-6-2014, Aalborg University
    % 29-11-2014, R. Olsen/M. Kemal, Aalborg University (Simulink)
    % 20-06-2015, F. Iov/M. Kemal, Aalborg University (Simulink toolbox for OPAL)
    
                % Input:
            %   - s [w/m^2], is the solar irradiance.
            %   - v [V], is the voltage at the connection point.
            %   - dP [PU], is the reference to active power change (curtailment).
            %   - dPlim [PU], is the reference to derated power (derate)
            %   - qRef [VAR], is the reactive power reference.
            %   - vRef [V], is the voltage reference.
            %
            % Output:
            %   - p [W], is the active power output
            %   - q [VAR], is the reactive power output
            %   - pAva [W], is the available power

            
           
        %properties
        param.vBase = 400;                % Voltage base [V].
        param.pRated = 6e3;               % Rated output power [W].
        param.sMax = 6e3;                 % Maximum apparent power [VA].
        param.A = 25;                     % Area of PV cell [m^2].
        param.eta = 0.25;                  % Efficency of cell [-].
        param.PF = 1;                     % Power factor [-].
        param.Ts = 60;                    % Sampling time (set to 0 if not used)

     %variable properties     
     persistent var;
     if isempty(var) 
        var.t_c = 0;                    %Time of caching
        var.p_c = 0;                    %Cached values
        var.q_c = 0;
        var.pAva_c = 0;
        var.kPV = 0;               % Gain from s to p [-].
        var.Qmode = 0;                  % Reactive power control mode [-].         
     end

        
        
% Solar to power conversion factor
     var.kPV = param.eta*param.A;
     
           if (param.Ts>0)
               if (time>(var.t_c+param.Ts))
                   [p,q,pAva,varNew] = samplePV(param,var,solarIrr,vMeas,dP,dPlim,qRef,vRef);
                   var=varNew;
                   var.p_c=p;
                   var.q_c=q;
                   var.pAva_c=pAva;
                   var.t_c=time;
                   var.Qmode = qMode;
               end
               p=var.p_c;
               q=var.q_c;
               pAva=var.pAva_c;
            else
               [p,q,pAva,varNew] = samplePV(param,var,solarIrr,vMeas,dP,dPlim,qRef,vRef);
               var=varNew;
               var.Qmode = qMode;
            end    

    
    
            
  end

== matlab function DiSC_ToolboxOpal_V12/SolarIrradiance/MATLAB Function ==
  data: day input; cc input; Go output; time input
function Go = SolarIrradianceDO(day,cc,time)
%#codegen
    %solarIrradianceS implements a solar irradiance model using
   %MATLAB embedded block of simulink for OPAL-RT
    %   The solar irradiance model can be used to investigate the behavior
    %   of e.g., photovoltaic systems. The model is based on the work by
    %   Heinriich Morf (1998-2013) and the book: "An Introduction to Solar
    %   Radiation", 1983.
    %   
    %
    % Revision
    % R. Pedersen 11-6-2014, Aalborg University
    % 29-11-2014, R. Olsen/M. Kemal, Aalborg University (Simulink)

            % Input:
            %   k [-], is the sample number. Used for zenit angle
            %   day [-], is the Julian day of the year (1-365)
            %   cc [-], is cloud cover (0-1);
            %
            % Output:
            %   Go [w/m^2], is the irradiance on a horizontal surface.    
     %parameter properties
        param.lat = 57;       % [degree], latitude of location (57 = Aalborg)
        param.t = 0.75;       % [-], Transmittance
        param.p = 100;        % [Kpa], Air pressure
        param.Ts = 60;        % [sec], sampling time
        
        % Parameters based on data and system identification
        param.a = 0.221;      % [-], Ångström-Prescott parameter
        param.b = 0.667;      % [-], Ångström-Prescott parameter
        param.tau = 0.25;     % [-], Transmission factor of irradiance through clouds 
        
        param.LPtau = 20;     % low-pass filter time constant [sec]
        param.WFT = 60;       % window filter window [sec]
       
     %variable properties     
     persistent var;
     if isempty(var)       
        % For filters
        var.LPyOld = 0;             % [-], place holder for low-pass filter
        var.WFyOld = 0;             % [-], place holder for window filter output
        var.WFuOld = zeros(1,40);   % [-], place holder for window filter input     end   
     end
            
            % Implement algorithm. Calculate y as a function of
            [Go,varNew] = sampleSIrr(param,var,time,day,cc);
            var=varNew;

end

== matlab function DiSC_ToolboxOpal_V12/Wind Turbine/MATLAB Function ==
  data: p output; wind input; vMeas input; dP input; dPlim input; qRef input; qMode input; vRef input; time input; q output; pAva output
function [p,q,pAva] = wtAssetSDO(wind,vMeas,dP,dPlim,qRef,qMode,vRef, time)
%#codegen
    %wtAssetS implements a simple P,Q controllable wind turbine system for Simulink.
    % This model works for Simulink and requires generatedWindFiles to
    % have been executed before running the simulink model
    % 
    %   The wtAsset can be set to follow an active power reference, output
    %   maximum power available or curtail power. It can also, at the same
    %   time be set to follow a reactive power reference, output the
    %   minimum reactive power according to the power factor or try to keep
    %   a voltage reference in the coupling point by controlling reactive
    %   power output.
    %   
    %   The model is partly based on the book
    %   "Optimal Control of Wind Energy Systems 2008".
    %   
    %   
    % Revision:
    % 23-05-2014, C. E. Sloth and R. Pedersen, Aalborg University. Notes:
    % 29-11-2014, R. Olsen/M. Kemal, Aalborg University (Simulink)
         %Parameters
        param.vBase = 20e3;               % Voltage base [V].
        param.pRated = 100e3;               % Rated output power [W].
        param.sMax = 100e3;                 % Maximum apparent power [VA].
        param.wMin = 3;                   % Cut-in wind speed [m/s].
        param.wMax = 25;                  % Cut-out wind speed [m/s].
        param.wRated = 12;                % Rated wind speed [m/s].
        param.rfTau = 20;                 % Time constant of rotor filter [s].
        param.PF = 1;                     % Power factor [-].
        param.Ts = 60;                    % Sampling time [sec].  

     %variables 
     persistent var;
     if isempty(var)         
        var.p_c=0;                      %All used for caching in between sampling period
        var.q_c=0;
        var.pAva_c=0;
        var.t_c=0;
        var.pOld = 0;                   % [w]. Place holder for the rotor initia filter
        
        var.avgFilterTime = 10*60;      % [s]. Time that the filter should look back 
        var.avgFilterBuf = zeros(ceil(10*60/60),1);
        var.Qmode = 0;                  % [-]. Reactive power control mode
        var.kWT = 3e6/(12^3);           % [-]. Gain from w^3 to p
     end

            % Power conversion constant
            var.kWT = param.pRated/(param.wRated^3);    
            
            % Implement algorithm. 
            
            if (param.Ts>0)
               if (time>(var.t_c+param.Ts))
                   [p,q,pAva,varNew] = sampleWT(param,var,wind,vMeas,dP,dPlim,qRef,vRef);
                   varNew.p_c=p;
                   varNew.q_c=q;
                   varNew.pAva_c=pAva;
                   varNew.t_c=time;
                   varNew.Qmode = qMode;
                   var=varNew;
               end
               p=var.p_c;
               q=var.q_c;
               pAva=var.pAva_c;
            else
                [p,q,pAva,varNew] = sampleWT(param,var,wind,vMeas,dP,dPlim,qRef,vRef);
                var=varNew;
            end
            
        
            
%          [p,q,pAva,varNew] = sampleWT(obj,var,wind,vMeas,dP,dPlim,qRef,vRef);
         
         
end

== matlab function DiSC_ToolboxOpal_V12/ControllableSwitch/MATLAB Function ==
  data: state output; uRef input; y output; day input; t input
function [state,y] = swAssetDO(uRef,day,t)
%#codegen
    % A Simulink implementation of swAsset using embedded MATLAB function
    %%swAsset implements a controllable switch.
    %   The swAsset can change the switch position between open and closed.
    %   The switch is used to change the electrical grid topology.
    %   To ensure realistic simulation scenarios a minimum time between
    %   switch state change has been incorporated, along with a maximum
    %   number of state changes per day.
    %   
    %   The model is intended for studying voltage control problems and
    %   power loss minimization. The switch works by inserting an
    %   admittance into the admittance matrix whenever the switch state is
    %   closed.
    %   
    % R. Pedersen 05-9-2014, Aalborg University
    % 20-06-2015, F. Iov/M. Kemal, Aalborg University (Simulink toolbox for OPAL)
    % This template includes the minimum set of functions required
    % to define a System object with discrete state.
    
    
            % Input:
            %   - uRef [-], is the reference to switch state (0=open, 1=closed).
            %   - k [-], is the sample.
            %   - day [-], is the day of the simulation (1-365).
            %
            % Output:
            %   - state [-], is the state of the switch, either open or closed.
            %   - y [-], is the admittance to be put into the grid admittance matrix.
            
            % If day changes reset the number of switches a day
            
            
            %parameters
            
        obj.zBase = 8;          % Base impedance of the grid [Ohm].              
        obj.Z = 1;              % Switch impedance [Ohm].        
        obj.Y = 1;              % Admittance of switch [S].        
        obj.Ts = 60;            % Sampling time [s].        
        obj.onPU = false;       % Indicates if the switch is used to simulate a system on per unit basis. true = yes, false = no [-]. 
        obj.nSwPrDay = 10;      % Maximum number of switch state changes per day [-].        
        obj.tMin = 10*60;       % Minimum time between switch position changes [s].         
        obj.kMin = 10;          % Minimum number of samples between switch position changes [-].         
        obj.swChOk = 1;         % Flag indicating if switch state can be changed (1=yes, 0=no [-]. )         
        
        
        %variables 
        persistent var;
        if isempty(var)  
         var.swState = 0;        % Switch state (0=open, 1=closed) [-].        
         var.swChDay = 0;        % Number of switch state changes that has occured in a day [-].         
         var.dayOld = -1;        % Used to check if day has changed [-].         
         var.swTimer = 0;        % Timer indicating if switch state change is allowed, i.e., the timer must be greater than kMin to apply change [-]. 
         var.state_c=0;      %All used for caching in between sampling period
         var.y_c=0;
         var.t_c=0;
         var.k=0; 
         var.swChOk = 1;         % Flag indicating if switch state can be changed (1=yes, 0=no [-]. )  
        end
        
             % Check if simulation is on PU
             if obj.onPU == true
                 obj.Z = obj.Z/obj.zBase;
             else
                 obj.Z = obj.Z;
             end
                 obj.Y = 1/obj.Z;
            
             % Compute minimum samples until switch state change
             obj.kMin = ceil(obj.tMin/obj.Ts);

            % Implement algorithm. 
            
            if (obj.Ts>0)
               if (t>(var.t_c+obj.Ts))
                   [state,y,varNew] = sampleSW(obj,var,uRef,var.k,day);
                   var=varNew;
                   var.state_c=state;
                   var.y_c=y;
                   var.t_c=t;
                   var.k=var.k+1;
                   
               end
               state=var.state_c;
               y=var.y_c;             
            else
                [state,y,varNew] = sampleSW(obj,var,uRef,var.k,day);
                var=varNew;
                var.k=var.k+1;
            
            end
            
          
end

== matlab function DiSC_ToolboxOpal_V12/scAsset/MATLAB Function ==
  data: v input; q output; qRef input; vRef input; t input
function q =scAssetDO(v,qRef,vRef,t)
%#codegen
    % A Simulink model of SC Asset using MATLAB embedded function block of simulink 
    % %scAsset implements a simple controllable static compensator asset.
    %   The scAsset can be set to inject or consume reactive power based
    %   on a reference  or do voltage droop control.
    %   
    %   This model is based on a simple algebraic principle, as it is
    %   intended for sampling times higher than 1 second.
    %   
    % Revision:
    % 23-06-2014, R. Pedersen, Aalborg University. Notes:
    % 29-11-2014, R. Olsen/M. Kemal, Aalborg University (Simulink)
    % 20-06-2015, F. Iov/M. Kemal, Aalborg University (Simulink toolbox for OPAL)
    
                % Input:
            %   - v [V], is the voltage magnitude on the bus.
            %   - qRef [VAR], is the reference to reactive power.
            %   - vRef [V], is the voltage reference.
            %
            % Output:
            %   - q [VAR], reactive power output.

    % parameter properties
        param.sBase = 10e3;             % Complex power base [VA].   
        param.vBase = 400;              % Voltage base [V].  
        param.qRatedMax = 10e3;         % Rated reactive power output [VAR].   
        param.qRatedMin = -10e3;        % Rated reactive power consumption [VAR].  
        param.Qmode = 0;                % Reactive power control mode [-].   
        param.onPU = false;             % Indicates if the static compensator is used to simulate a system on per unit basis. true = yes, false = no [-]. 
        param.Ts=60;                    % Sample time [s]
        
        
        %variables
       persistent var;
       if isempty(var);
           
       var.t_c=0;  %Caching time
       var.q_c=0;  %Cached q value
       var.k=0;
           
       end

            % Implement algorithm. 
                        
             if (param.Ts>0)
               if (t>(var.t_c+param.Ts))
                   var.q_c = sampleSC(param,v,qRef,vRef);
                   var.t_c=t;
                   var.k=var.k+1;
               end
               q=var.q_c;
            else
                q = sampleSC(param,v,qRef,vRef);
                var.k=var.k+1;
             end     
  
         

    
end
